simulink model "SR25"  (R2024a)
settings: Solver=FixedStepDiscrete  StartTime=0.0  StopTime=5  FixedStep=0.01  RelTol=1e-3  EnableMultiTasking=on
PreLoadFcn:
  | try, model_open; catch, disp('Error occurred while executing model pre-load callback: model_open.m'); disp('Please assure that the MATLAB working directory is set to the model directory before opening.'); end
InitFcn:
  | try, model_open; catch, end
undefined symbols (not defined in the file or in its folder): dt, GCM, raptor_get_safe_string, raptor_xcp_function
libraries: Raptor_lib x40, Utilities x13, TireTemperature x12, simulink x5, IO x5, APPS_BSPC x4, RotorTemperature x4, FlowRate x3, Cooling x2, BMS x2, Brakes x2, StateMachine x2
(part 3 of 3)

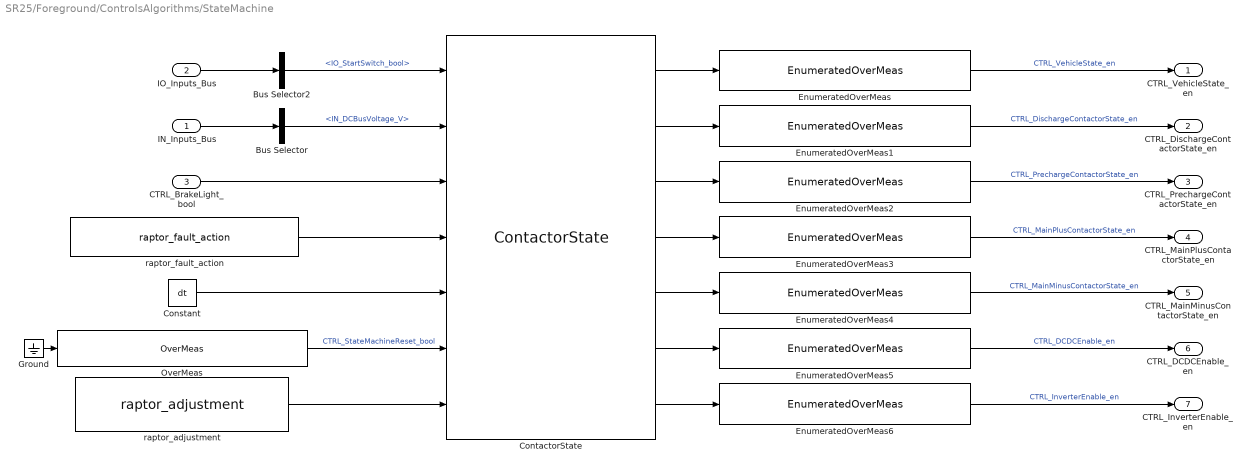
== system SR25/Foreground/ControlsAlgorithms/StateMachine ==
  IN_Inputs_Bus : Inport
  IO_Inputs_Bus : Inport  Port=2
  CTRL_BrakeLight_bool : Inport  Port=3
  Bus Selector : BusSelector  OutputSignals=IN_PM100DX_Bus.IN_DCBusVoltage_V
  Bus Selector2 : BusSelector  OutputSignals=IO_DigitalInputs_Bus.IO_StartSwitch_bool
  Constant : Constant  Value=dt
  ContactorState : StateMachine/ContactorState  SystemSampleTime=-1  VariantActivationTime=update diagram  AllowFlexibleInterface=on  Latency=0  AutoFrameSizeCalculation=off
  EnumeratedOverMeas : Utilities/EnumeratedOverMeas  sigName='CTRL_VehicleState_en'  enumName='VehicleState'
  EnumeratedOverMeas1 : Utilities/EnumeratedOverMeas  sigName='CTRL_DischargeContactorState_en'  enumName='ContactorState'
  EnumeratedOverMeas2 : Utilities/EnumeratedOverMeas  sigName='CTRL_PrechargeContactorState_en'  enumName='ContactorState'
  EnumeratedOverMeas3 : Utilities/EnumeratedOverMeas  sigName='CTRL_MainPlusContactorState_en'  enumName='ContactorState'
  EnumeratedOverMeas4 : Utilities/EnumeratedOverMeas  sigName='CTRL_MainMinusContactorState_en'  enumName='ContactorState'
  EnumeratedOverMeas5 : Utilities/EnumeratedOverMeas  sigName='CTRL_DCDCEnable_en'  enumName='DCDCStatus'
  EnumeratedOverMeas6 : Utilities/EnumeratedOverMeas  sigName='CTRL_InverterEnable_en'  enumName='InverterStatus'
  Ground : Ground
  OverMeas : Utilities/OverMeas  sigName='CTRL_StateMachineReset_bool'  minimum=0  maximum=1
  raptor_adjustment : Raptor_lib/Data Storage/raptor_adjustment  paramName='CTRL_PrechargeThresh_V'  nameSource=Parameter  initValue=288  dataType=double  storage=Calibration  calDispType=Number  calEnum={'False', 'True'}  calGain=1.0  calOffset=0.0  calMax=inf  calMin=-inf  calFormat='-1'  calUnit=''  calHelp=''  calAccess=1  calFunction=raptor_xcp_function(gcb)  calDispHeaders=off  calColHeaders={'Col1' 'Col2' 'Col3'}  calRowHeaders={'Row1' 'Row2' 'Row3'}
      settings: SourceProductName=Raptor
  raptor_fault_action : Raptor_lib/Faults/raptor_fault_action  actionName='VehicleFault'  calVisible=on  calAccess=1  calFunction='System | FaultManager | FaultAction'
      settings: SourceProductName=Raptor
  CTRL_VehicleState_en : Outport
  CTRL_DischargeContactorState_en : Outport  Port=2
  CTRL_PrechargeContactorState_en : Outport  Port=3
  CTRL_MainPlusContactorState_en : Outport  Port=4
  CTRL_MainMinusContactorState_en : Outport  Port=5
  CTRL_DCDCEnable_en : Outport  Port=6
  CTRL_InverterEnable_en : Outport  Port=7
  wires:
  IN_Inputs_Bus/1 -> Bus Selector/1
  ContactorState/1 -> EnumeratedOverMeas/1
  ContactorState/2 -> EnumeratedOverMeas1/1
  ContactorState/3 -> EnumeratedOverMeas2/1
  ContactorState/4 -> EnumeratedOverMeas3/1
  ContactorState/5 -> EnumeratedOverMeas4/1
  EnumeratedOverMeas/1 -> CTRL_VehicleState_en/1  "CTRL_VehicleState_en"
  EnumeratedOverMeas1/1 -> CTRL_DischargeContactorState_en/1  "CTRL_DischargeContactorState_en"
  EnumeratedOverMeas2/1 -> CTRL_PrechargeContactorState_en/1  "CTRL_PrechargeContactorState_en"
  EnumeratedOverMeas3/1 -> CTRL_MainPlusContactorState_en/1  "CTRL_MainPlusContactorState_en"
  EnumeratedOverMeas4/1 -> CTRL_MainMinusContactorState_en/1  "CTRL_MainMinusContactorState_en"
  Constant/1 -> ContactorState/5
  IO_Inputs_Bus/1 -> Bus Selector2/1
  CTRL_BrakeLight_bool/1 -> ContactorState/3
  Bus Selector/1 -> ContactorState/2  "<IN_DCBusVoltage_V>"
  ContactorState/6 -> EnumeratedOverMeas5/1
  EnumeratedOverMeas5/1 -> CTRL_DCDCEnable_en/1  "CTRL_DCDCEnable_en"
  ContactorState/7 -> EnumeratedOverMeas6/1
  EnumeratedOverMeas6/1 -> CTRL_InverterEnable_en/1  "CTRL_InverterEnable_en"
  OverMeas/1 -> ContactorState/6  "CTRL_StateMachineReset_bool"
  Ground/1 -> OverMeas/1
  Bus Selector2/1 -> ContactorState/1  "<IO_StartSwitch_bool>"
  raptor_fault_action/1 -> ContactorState/4
  raptor_adjustment/1 -> ContactorState/7

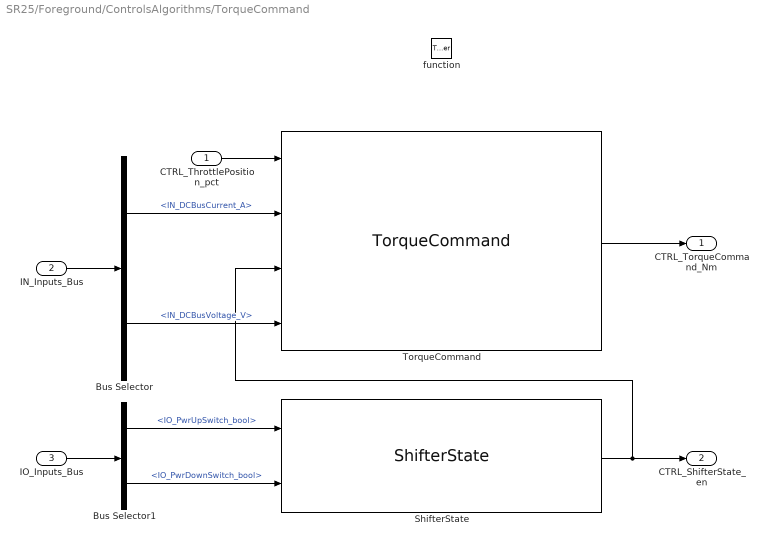
== system SR25/Foreground/ControlsAlgorithms/TorqueCommand ==
  CTRL_ThrottlePosition_pct : Inport
  IN_Inputs_Bus : Inport  Port=2
  IO_Inputs_Bus : Inport  Port=3
  function : TriggerPort  TriggerType=function-call  VariantControl=(inherit)
  Bus Selector : BusSelector  OutputSignals=IN_PM100DX_Bus.IN_DCBusCurrent_A,IN_PM100DX_Bus.IN_DCBusVoltage_V
  Bus Selector1 : BusSelector  OutputSignals=IO_DigitalInputs_Bus.IO_PwrUpSwitch_bool,IO_DigitalInputs_Bus.IO_PwrDownSwitch_bool
  ShifterState : TorqueCommand/ShifterState  SystemSampleTime=-1  VariantActivationTime=update diagram  AllowFlexibleInterface=on  Latency=0  AutoFrameSizeCalculation=off
  TorqueCommand : TorqueCommand/TorqueCommand  SystemSampleTime=-1  VariantActivationTime=update diagram  AllowFlexibleInterface=on  Latency=0  AutoFrameSizeCalculation=off
  CTRL_TorqueCommand_Nm : Outport
  CTRL_ShifterState_en : Outport  Port=2
  wires:
  CTRL_ThrottlePosition_pct/1 -> TorqueCommand/1
  IN_Inputs_Bus/1 -> Bus Selector/1
  IO_Inputs_Bus/1 -> Bus Selector1/1
  Bus Selector1/1 -> ShifterState/1  "<IO_PwrUpSwitch_bool>"
  Bus Selector1/2 -> ShifterState/2  "<IO_PwrDownSwitch_bool>"
  ShifterState/1 -> CTRL_ShifterState_en/1, TorqueCommand/3
  TorqueCommand/1 -> CTRL_TorqueCommand_Nm/1
  Bus Selector/1 -> TorqueCommand/2  "<IN_DCBusCurrent_A>"
  Bus Selector/2 -> TorqueCommand/4  "<IN_DCBusVoltage_V>"

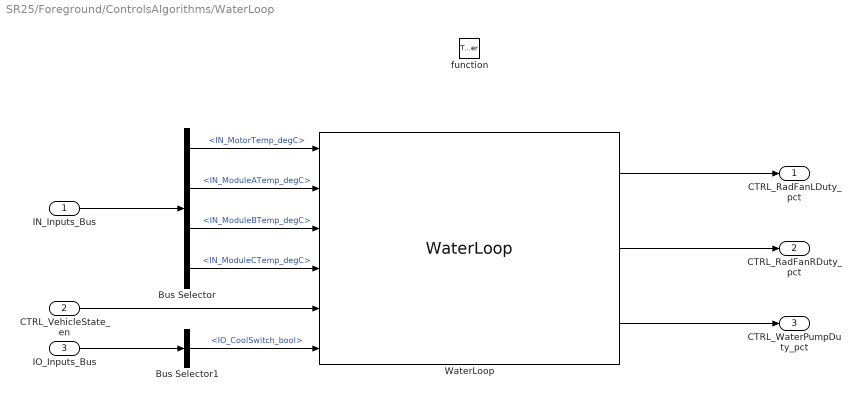
== system SR25/Foreground/ControlsAlgorithms/WaterLoop ==
  IN_Inputs_Bus : Inport
  CTRL_VehicleState_en : Inport  Port=2
  IO_Inputs_Bus : Inport  Port=3
  function : TriggerPort  TriggerType=function-call  VariantControl=(inherit)
  Bus Selector : BusSelector  OutputSignals=IN_PM100DX_Bus.IN_MotorTemp_degC,IN_PM100DX_Bus.IN_ModuleATemp_degC,IN_PM100DX_Bus.IN_ModuleBTemp_degC,IN_PM100DX_Bus.IN_ModuleCTemp_degC
  Bus Selector1 : BusSelector  OutputSignals=IO_DigitalInputs_Bus.IO_CoolSwitch_bool
  WaterLoop : Cooling/WaterLoop  SystemSampleTime=-1  VariantActivationTime=update diagram  AllowFlexibleInterface=on  Latency=0  AutoFrameSizeCalculation=off
  CTRL_RadFanLDuty_pct : Outport
  CTRL_RadFanRDuty_pct : Outport  Port=2
  CTRL_WaterPumpDuty_pct : Outport  Port=3
  wires:
  IN_Inputs_Bus/1 -> Bus Selector/1
  CTRL_VehicleState_en/1 -> WaterLoop/5
  Bus Selector/4 -> WaterLoop/4  "<IN_ModuleCTemp_degC>"
  Bus Selector/3 -> WaterLoop/3  "<IN_ModuleBTemp_degC>"
  Bus Selector/2 -> WaterLoop/2  "<IN_ModuleATemp_degC>"
  Bus Selector/1 -> WaterLoop/1  "<IN_MotorTemp_degC>"
  IO_Inputs_Bus/1 -> Bus Selector1/1
  Bus Selector1/1 -> WaterLoop/6  "<IO_CoolSwitch_bool>"
  WaterLoop/1 -> CTRL_RadFanLDuty_pct/1
  WaterLoop/2 -> CTRL_RadFanRDuty_pct/1
  WaterLoop/3 -> CTRL_WaterPumpDuty_pct/1

== system SR25/Foreground/IO/Inputs ==
  AnalogInputs : IO/AnalogInputs  SystemSampleTime=-1  VariantActivationTime=update diagram  AllowFlexibleInterface=on  Latency=0  AutoFrameSizeCalculation=off
  Bus Creator : BusCreator  Inputs=24
  Bus Creator1 : BusCreator  Inputs=3
  Bus Creator2 : BusCreator  Inputs=7
  Bus Creator3 : BusCreator  Inputs=2
  CANInputs : IO/CANInputs  SystemSampleTime=-1  VariantActivationTime=update diagram  AllowFlexibleInterface=on  Latency=0  AutoFrameSizeCalculation=off
  DigitalInputs : IO/DigitalInputs  SystemSampleTime=-1  VariantActivationTime=update diagram  AllowFlexibleInterface=on  Latency=0  AutoFrameSizeCalculation=off
  IO_Inputs_Bus : Outport
  wires:
  AnalogInputs/2 -> Bus Creator/2
  AnalogInputs/1 -> Bus Creator/1
  Bus Creator/1 -> Bus Creator1/1  "IO_AnalogInputs_Bus"
  Bus Creator1/1 -> IO_Inputs_Bus/1  "IO_Inputs_Bus"
  DigitalInputs/1 -> Bus Creator2/1
  DigitalInputs/2 -> Bus Creator2/2
  DigitalInputs/3 -> Bus Creator2/3
  DigitalInputs/4 -> Bus Creator2/4
  Bus Creator2/1 -> Bus Creator1/2  "IO_DigitalInputs_Bus"
  AnalogInputs/3 -> Bus Creator/3
  AnalogInputs/4 -> Bus Creator/4
  AnalogInputs/5 -> Bus Creator/5
  AnalogInputs/6 -> Bus Creator/6
  AnalogInputs/7 -> Bus Creator/7
  AnalogInputs/8 -> Bus Creator/8
  AnalogInputs/9 -> Bus Creator/9
  AnalogInputs/10 -> Bus Creator/10
  AnalogInputs/11 -> Bus Creator/11
  AnalogInputs/12 -> Bus Creator/12
  CANInputs/1 -> Bus Creator3/1
  CANInputs/2 -> Bus Creator3/2
  Bus Creator3/1 -> Bus Creator1/3  "IO_CANInputs_Bus"
  DigitalInputs/5 -> Bus Creator2/5
  AnalogInputs/13 -> Bus Creator/13
  AnalogInputs/14 -> Bus Creator/14
  AnalogInputs/15 -> Bus Creator/15
  AnalogInputs/16 -> Bus Creator/16
  AnalogInputs/17 -> Bus Creator/17
  AnalogInputs/18 -> Bus Creator/18
  AnalogInputs/19 -> Bus Creator/19
  AnalogInputs/20 -> Bus Creator/20
  AnalogInputs/21 -> Bus Creator/21
  AnalogInputs/22 -> Bus Creator/22
  AnalogInputs/23 -> Bus Creator/23
  AnalogInputs/24 -> Bus Creator/24
  DigitalInputs/6 -> Bus Creator2/6
  DigitalInputs/7 -> Bus Creator2/7

== system SR25/Foreground/IO/Outputs ==
  IO_Outputs_Bus : Inport
  Bus Selector : BusSelector  OutputSignals=IO_DigitalOutputs_Bus,IO_CANOutputs_Bus
  CANOutputs : IO/CANOutputs  SystemSampleTime=-1  VariantActivationTime=update diagram  AllowFlexibleInterface=on  Latency=0  AutoFrameSizeCalculation=off
  DigitalOutputs : IO/DigitalOutputs  SystemSampleTime=-1  VariantActivationTime=update diagram  AllowFlexibleInterface=on  Latency=0  AutoFrameSizeCalculation=off
  wires:
  IO_Outputs_Bus/1 -> Bus Selector/1
  Bus Selector/1 -> DigitalOutputs/1  "<IO_DigitalOutputs_Bus>"
  Bus Selector/2 -> CANOutputs/1  "<IO_CANOutputs_Bus>"

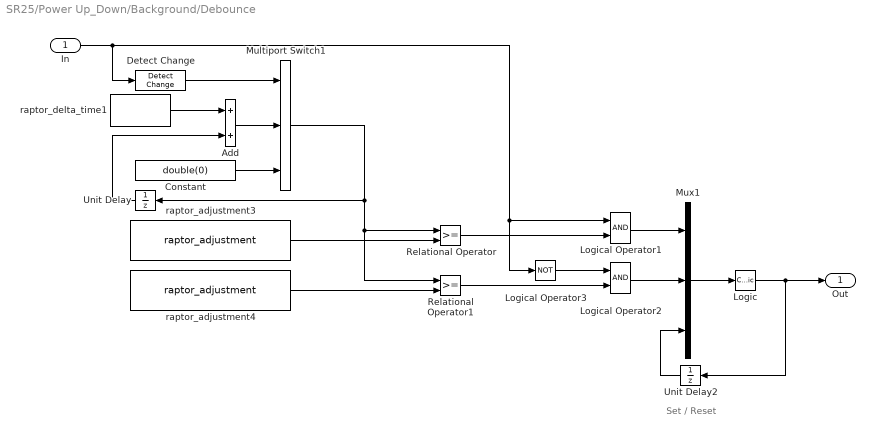
== system SR25/Power Up_Down/Background/Debounce ==
  note: Set / Reset
  In : Inport
  Add : Sum
  Constant : Constant  Value=double(0)
  Detect Change : simulink/Logic and Bit Operations/Detect Change  vinit=0  OutDataTypeStr=boolean
  Logic : CombinatorialLogic  TruthTable=[0;1;0;0;1;1;0;0]
  Logical Operator1 : Logic  AllPortsSameDT=off  OutDataTypeStr=boolean
  Logical Operator2 : Logic  AllPortsSameDT=off  OutDataTypeStr=boolean
  Logical Operator3 : Logic  Operator=NOT  Inputs=1  AllPortsSameDT=off  OutDataTypeStr=boolean
  Multiport Switch1 : MultiPortSwitch  DataPortOrder=Zero-based contiguous  Inputs=2  zeroidx=on  SaturateOnIntegerOverflow=off  InputSameDT=off
  Mux1 : Mux  Inputs=3
  Relational Operator : RelationalOperator  OutDataTypeStr=boolean  InputSameDT=off
  Relational Operator1 : RelationalOperator  OutDataTypeStr=boolean  InputSameDT=off
  Unit Delay : UnitDelay  SampleTime=-1  HasFrameUpgradeWarning=on
  Unit Delay2 : UnitDelay  InitialCondition=1  SampleTime=-1  HasFrameUpgradeWarning=on
  raptor_adjustment3 : Raptor_lib/Data Storage/raptor_adjustment  paramName='KeySwHiTimeThr'  nameSource=Parameter  initValue=0.2  dataType=double  storage=Calibration  calDispType=Number  calEnum={'Active Low', 'Active High'}  calGain=1  calOffset=0  calMax=inf  calMin=-inf  calFormat='-1'  calUnit='sec'  calHelp='State high time threshold'  calAccess=1  calFunction=group  calDispHeaders=off  calColHeaders={'Col1' 'Col2' 'Col3'}  calRowHeaders={'Row1' 'Row2' 'Row3'}
      settings: SourceProductName=Raptor
  raptor_adjustment4 : Raptor_lib/Data Storage/raptor_adjustment  paramName='KeySwLoTimeThr'  nameSource=Parameter  initValue=0.2  dataType=double  storage=Calibration  calDispType=Number  calEnum={'Active Low', 'Active High'}  calGain=1  calOffset=0  calMax=inf  calMin=-inf  calFormat='-1'  calUnit='sec'  calHelp='State low time threshold'  calAccess=1  calFunction=group  calDispHeaders=off  calColHeaders={'Col1' 'Col2' 'Col3'}  calRowHeaders={'Row1' 'Row2' 'Row3'}
      settings: SourceProductName=Raptor
  raptor_delta_time1 : Raptor_lib/Triggers/raptor_delta_time  unit=seconds
      settings: SourceProductName=Raptor
  Out : Outport  VectorParamsAs1DForOutWhenUnconnected=off
  wires:
  Detect Change/1 -> Multiport Switch1/1
  Logical Operator3/1 -> Logical Operator2/1
  Relational Operator/1 -> Logical Operator1/2
  Logical Operator2/1 -> Mux1/2
  Logical Operator1/1 -> Mux1/1
  Mux1/1 -> Logic/1
  Unit Delay2/1 -> Mux1/3
  In/1 -> Detect Change/1, Logical Operator1/1, Logical Operator3/1
  Multiport Switch1/1 -> Unit Delay/1, Relational Operator/1, Relational Operator1/1
  Add/1 -> Multiport Switch1/2
  Constant/1 -> Multiport Switch1/3
  Relational Operator1/1 -> Logical Operator2/2
  Logic/1 -> Unit Delay2/1, Out/1
  Unit Delay/1 -> Add/2
  raptor_delta_time1/1 -> Add/1
  raptor_adjustment4/1 -> Relational Operator1/2
  raptor_adjustment3/1 -> Relational Operator/2

== system SR25/Power Up_Down/Background/Raise Shutdown Event ==
  Trigger : TriggerPort  TriggerType=falling  VariantControl=Variant
  Constant : Constant  Value=boolean(1)
  Function-Call Generator : simulink/Ports & Subsystems/Function-Call Generator  sample_time=-1  numberOfIterations=1  DisallowWideOutput=off
  raptor_data_def : Raptor_lib/Data Storage/raptor_data_def  dataName='FgndTasksStopped'  initValue=0  dataType=boolean  storage=Volatile (RAM)  calVisible=on  calType=Measurement  calDispType=Number  calEnum={'False', 'True'}  calGain=1.0  calOffset=0  calMin=-Inf  calMax=Inf  calFormat='-1'  calUnit='Bool'  calHelp='Boolean indicating foreground tasks stopped'  calAccess=1  calFunction=group  calDispHeaders=off  calColHeaders={'Col1' 'Col2' 'Col3'}  calRowHeaders={'Row1' 'Row2' 'Row3'}
      settings: SourceProductName=Raptor
  raptor_data_write : Raptor_lib/Data Storage/raptor_data_write  dataName='FgndTasksStopped'  dataShape=Scalar  idxSource=Input Port  idxRow=1  idxCol=1
      settings: SourceProductName=Raptor
  raptor_shutdown : Raptor_lib/Triggers/raptor_shutdown  null=0
      settings: SourceProductName=Raptor
  wires:
  Constant/1 -> raptor_data_write/1
  Function-Call Generator/1 -> raptor_shutdown/Trigger

== system SR25/Power Up_Down/Background/Raise Startup Event ==
  Enable : EnablePort
  Trigger : TriggerPort  VariantControl=Variant
  Function-Call Generator : simulink/Ports & Subsystems/Function-Call Generator  sample_time=-1  numberOfIterations=1  DisallowWideOutput=off
  raptor_startup : Raptor_lib/Triggers/raptor_startup  null=0
      settings: SourceProductName=Raptor
  wires:
  Function-Call Generator/1 -> raptor_startup/Trigger

== system SR25/Power Up_Down/Background/Store EEPROM ==
  Trigger : TriggerPort  TriggerType=falling  VariantControl=Variant
  Function-Call Generator : simulink/Ports & Subsystems/Function-Call Generator  sample_time=-1  numberOfIterations=1  DisallowWideOutput=off
  raptor_store_nv : Raptor_lib/Data Storage/raptor_store_nv  null=0
      settings: SourceProductName=Raptor
  wires:
  Function-Call Generator/1 -> raptor_store_nv/Trigger
